simulink model "UDE_FINAL"  (R2021a)
settings: Solver=ode15s  StartTime=0.0  StopTime=10  FixedStep=0.001  RelTol=1e-3
values from neighbouring files (symbols this model uses):
  A = [0       1    0 ... (first row only)    [H_INFINITY_FINAL.m]    (also in UDE_CODE_FINAL.m)
  A_m = [0      1    0 ... (first row only)    [UDE_CODE_FINAL.m]
  A_plus_delA = A+del_A    [UDE_CODE_FINAL.m]
  B = [0 0 53.19]'    [UDE_CODE_FINAL.m]
  B_m = [0 0 -10000]'    [UDE_CODE_FINAL.m]
  B_plus = vv    [UDE_CODE_FINAL.m]
  C_m = [ 1 0 0]    [UDE_CODE_FINAL.m]
  kk = A_m-A    [UDE_CODE_FINAL.m]
settings Model: Creator=ANUPAM MISHRA  LastModifiedBy=ANIRUDH
settings SolverCC: AlgebraicLoopSolver=TrustRegion
settings DebuggingCC: SFMachineParentedDataDiag=warning

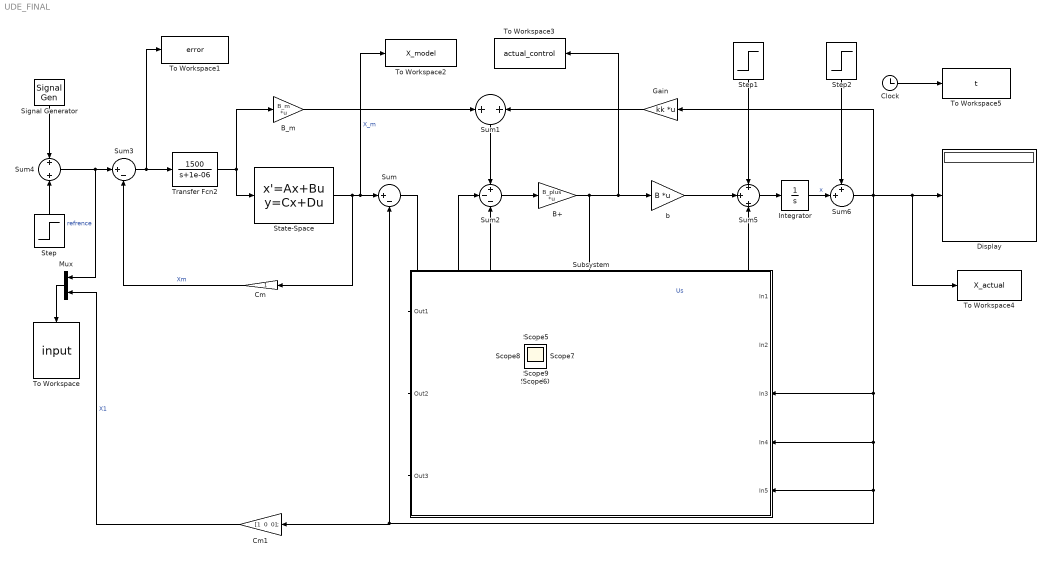
== system UDE_FINAL ==
  B+ : Gain  Gain=B_plus  Multiplication=Matrix(K*u)
  B_m : Gain  Gain=B_m  Multiplication=Matrix(K*u)
  Clock : Clock
      settings: Decimation=1
  Cm : Gain
  Cm1 : Gain  Gain="[1  0  0];"
  Display : Display
  Gain : Gain  Gain=kk  Multiplication=Matrix(K*u)
  Integrator : Integrator
  Mux : Mux  Inputs=2
  Signal Generator : SignalGenerator  Amplitude=2  Frequency=10
  State-Space : StateSpace  A=A_m  B=B_m  C=C_m  D=0  InitialCondition=0
  Step : Step  Time=0  After=4  SampleTime=0
  Step1 : Step  Time=2  After=[50 50 50]';  SampleTime=0
  Step2 : Step  Time=4  After=0.1  SampleTime=0
  Subsystem : Subsystem
  Sum : Sum  Inputs=|+-
  Sum1 : Sum
  Sum2 : Sum  Inputs=+--
  Sum3 : Sum  Inputs=|+-
  Sum4 : Sum  Inputs=+|+
  Sum5 : Sum  Inputs=+|+|+
  Sum6 : Sum  Inputs=++|
  To Workspace : ToWorkspace  VariableName=input  SaveFormat=Structure With Time  SampleTime=-1
  To Workspace1 : ToWorkspace  VariableName=error  SaveFormat=Structure With Time  SampleTime=-1
  To Workspace2 : ToWorkspace  VariableName=X_model  SaveFormat=Structure With Time  SampleTime=-1
  To Workspace3 : ToWorkspace  VariableName=actual_control  SaveFormat=Structure With Time  SampleTime=-1
  To Workspace4 : ToWorkspace  VariableName=X_actual  SaveFormat=Structure With Time  SampleTime=-1
  To Workspace5 : ToWorkspace  VariableName=t  SampleTime=-1
  Transfer Fcn2 : TransferFcn  Numerator=[1500]  Denominator=[1 1e-06]
  b : Gain  Gain=B  Multiplication=Matrix(K*u)
  Scope{,1..10} (11 alike) : Scope
  wires:
  State-Space/1 -> To Workspace2/1, Sum/1, Cm/1  "X_m"
  Sum3/1 -> To Workspace1/1, Transfer Fcn2/1
  Transfer Fcn2/1 -> State-Space/1, B_m/1
  Cm/1 -> Sum3/2  "Xm"
  B_m/1 -> Sum1/1
  Gain/1 -> Sum1/2
  Sum1/1 -> Sum2/1
  Sum2/1 -> B+/1
  Cm1/1 -> Mux/2  "X1"
  B+/1 -> To Workspace3/1, b/1, Subsystem/1(In1)  "Us"
  Sum5/1 -> Integrator/1
  Sum/1 -> Subsystem/2(In2)
  Subsystem/1(Out1) -> Sum5/3
  Subsystem/2(Out2) -> Sum2/2
  Subsystem/3(Out3) -> Sum2/3
  Signal Generator/1 -> Sum4/1
  Step/1 -> Sum4/2
  Sum4/1 -> Mux/1, Sum3/1  "refrence"
  Mux/1 -> To Workspace/1
  Clock/1 -> To Workspace5/1
  b/1 -> Sum5/2
  Step1/1 -> Sum5/1
  Integrator/1 -> Sum6/2  "x"
  Step2/1 -> Sum6/1
  Sum6/1 -> To Workspace4/1, Display/1, Subsystem/4(In4), Cm1/1, Sum/2, Subsystem/5(In5), Subsystem/3(In3), Gain/1

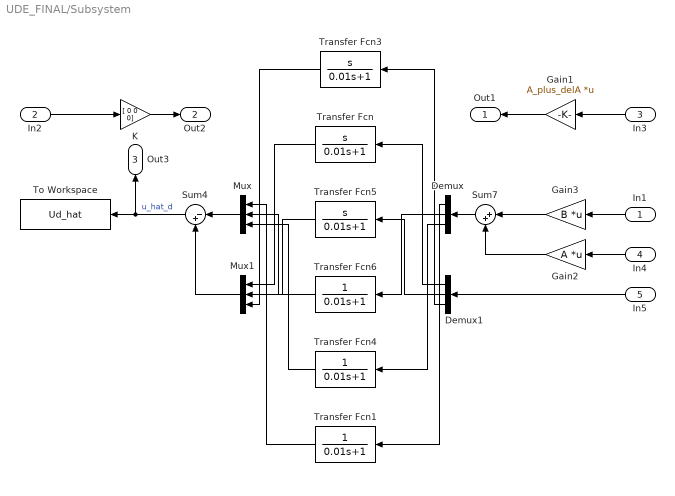
== system UDE_FINAL/Subsystem ==
  In1 : Inport
  In2 : Inport  Port=2
  In3 : Inport  Port=3
  In4 : Inport  Port=4
  In5 : Inport  Port=5
  Demux : Demux  Outputs=3
  Demux1 : Demux  Outputs=3
  Gain1 : Gain  Gain=A_plus_delA  Multiplication=Matrix(K*u)
  Gain2 : Gain  Gain=A  Multiplication=Matrix(K*u)
  Gain3 : Gain  Gain=B  Multiplication=Matrix(K*u)
  K : Gain  Gain="[ 0   0    0]"
  Mux : Mux  Inputs=3
  Mux1 : Mux  Inputs=3
  Sum4 : Sum  Inputs=|-+
  Sum7 : Sum  Inputs=|++
  To Workspace : ToWorkspace  VariableName=Ud_hat  SampleTime=-1
      settings: Save2DSignal=2-D array (concatenate along first dimension)
  Transfer Fcn : TransferFcn  Numerator="[  1  0]"  Denominator="[ 0.01    1]"
  Transfer Fcn1 : TransferFcn  Denominator="[ 0.01      1]"
  Transfer Fcn3 : TransferFcn  Numerator="[  1  0]"  Denominator="[ 0.01    1]"
  Transfer Fcn4 : TransferFcn  Denominator="[ 0.01      1]"
  Transfer Fcn5 : TransferFcn  Numerator="[  1  0]"  Denominator="[ 0.01    1]"
  Transfer Fcn6 : TransferFcn  Denominator="[ 0.01      1]"
  Out1 : Outport
  Out2 : Outport  Port=2
  Out3 : Outport  Port=3
  wires:
  Demux1/3 -> Transfer Fcn3/1
  Gain2/1 -> Sum7/2
  Demux1/1 -> Transfer Fcn/1
  Demux1/2 -> Transfer Fcn5/1
  In5/1 -> Demux1/1
  Transfer Fcn/1 -> Mux1/1
  Sum7/1 -> Demux/1
  Demux/2 -> Transfer Fcn6/1
  Transfer Fcn5/1 -> Mux1/2
  Gain1/1 -> Out1/1
  Demux/3 -> Transfer Fcn4/1
  Transfer Fcn4/1 -> Mux/3
  Gain3/1 -> Sum7/1
  Transfer Fcn6/1 -> Mux/2
  In1/1 -> Gain3/1
  K/1 -> Out2/1
  Mux1/1 -> Sum4/2
  Transfer Fcn3/1 -> Mux1/3
  Transfer Fcn1/1 -> Mux/1
  Demux/1 -> Transfer Fcn1/1
  Mux/1 -> Sum4/1
  Sum4/1 -> Out3/1, To Workspace/1  "u_hat_d"
  In2/1 -> K/1
  In4/1 -> Gain2/1
  In3/1 -> Gain1/1
